simulink model "simulation"  (R2021b)
settings: Solver=ode3  StartTime=0.0  StopTime=0.2  FixedStep=Ts  RelTol=1e-3
model workspace (MAT data in the model file):
  J_x = 8e-06
  J_y = 7.85e-06
  K0_x = 0.1
  K0_y = 0.1
  Kf_x = 0.00565
  Kf_y = 0.00553
  Ki_x = 0.00424
  Ki_y = 0.00406
  Kp_x = -0.1074
  Kp_y = -0.1545
  Kr_x = 1
  Kr_y = 1
  Kt_x = -931
  Kt_y = -914
  SNR = 1
  Ts = 1e-06
  aire_photodiode = 7.02
  angle_range = 15
  angle_x = 0
  angle_z = 0
  barcode_image = [92 38 38 38 38 38 38 38 38 38 38 38 ... (1616960 elements, 1304x1240)]
  fc_highpass = 300
  fc_transimpedance = 10000
  fini_surface = 0
  gain_filtre = 100
  gain_photodiode = 0.42
  gain_transimpedance = 1500000
  hauteur = 35
  largeur = 70
  lum_elec = 0.001
  lum_nat = 0.001
  noyau_gaussien = [0 0 0 0 0 0 0 0 0 0 0 0 ... (2601 elements, 51x51)]
  p_x = 0
  p_y = 0
  p_z = -100
  puissance_laser = 1
  pwm_freq = 30000
  pwm_period = 3e-05
  ratio_x = 0.0806451612903
  ratio_y = 0.0766871165644
  rayon = 0
  scan_freq = 15
  scan_period = 0.1
  seuil_comparateur = 1
  temps_echantillonnage = 5
  tolerance_decodage = 0.01
  v_range = 0.261799387799
libraries: simulink x5
(part 1 of 2)
settings Model: Creator=fredericmarcotte  LastModifiedBy=sammynoelparise

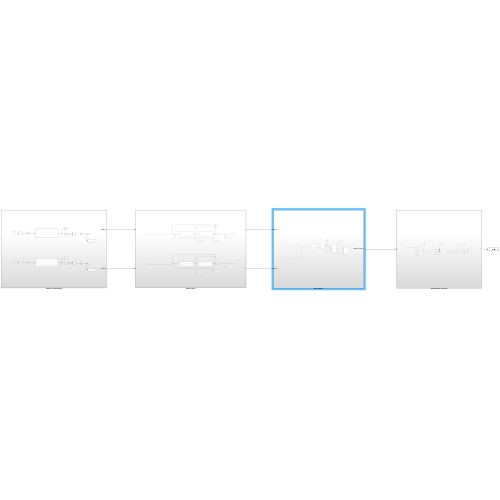
[thumbnail: Simulink's stored preview of the top-level diagram]
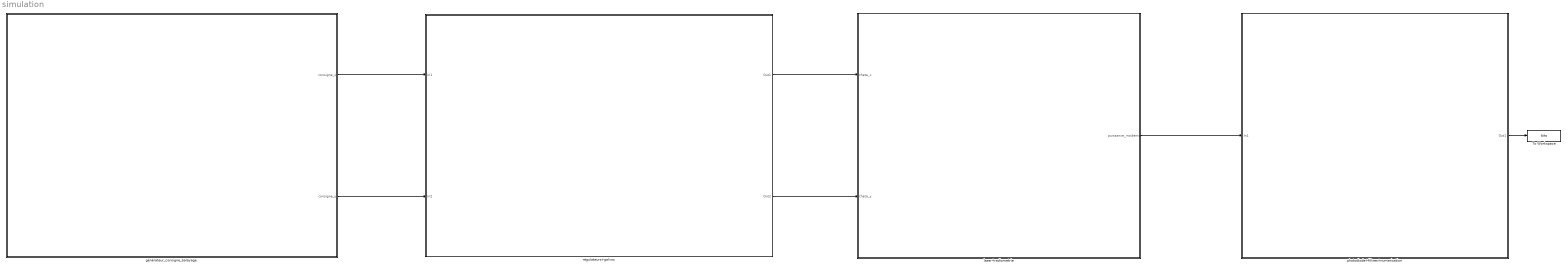
== system simulation ==
  To Workspace : ToWorkspace  VariableName=bits  SaveFormat=Timeseries  SampleTime=-1
  générateur_consigne_balayage : Subsystem
  laser+radiometrie : Subsystem
  photodiode+filtres+numerisation : Subsystem
  régulateurs+galvos : Subsystem
  wires:
  générateur_consigne_balayage/1(consigne_x) -> régulateurs+galvos/1(In1)
  générateur_consigne_balayage/2(consigne_y) -> régulateurs+galvos/2(In2)
  régulateurs+galvos/1(Out1) -> laser+radiometrie/1(theta_x)
  régulateurs+galvos/2(Out2) -> laser+radiometrie/2(theta_y)
  laser+radiometrie/1(puissance_incidente) -> photodiode+filtres+numerisation/1(In1)
  photodiode+filtres+numerisation/1(Out1) -> To Workspace/1
